simulink model "BacklashImplemented"  (R2018a)
settings: Solver=FixedStepDiscrete  StartTime=0.0  StopTime=10.0  RelTol=1e-3
settings Model: Creator=Laxman  LastModifiedBy=Laxman

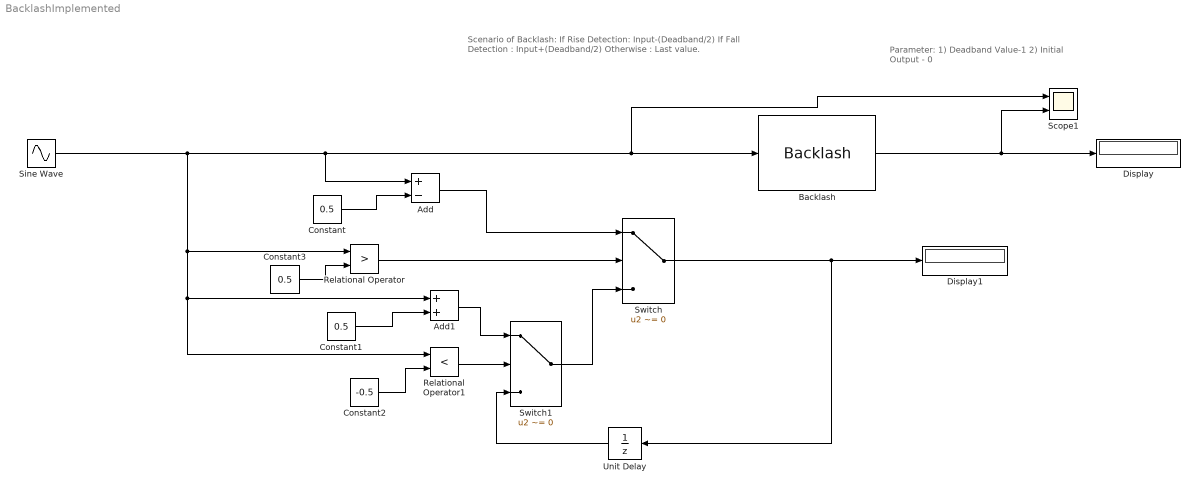
== system BacklashImplemented ==
  note: Parameter: 1) Deadband Value-1
      | 2) Initial Output - 0
  note: Scenario of Backlash:
      | If Rise Detection: Input-(Deadband/2)
      | If Fall Detection : Input+(Deadband/2)
      | Otherwise : Last value.
  Add : Sum  Inputs=+-
  Add1 : Sum
  Backlash : Backlash
  Constant : Constant  Value=0.5
  Constant1 : Constant  Value=0.5
  Constant2 : Constant  Value=-0.5
  Constant3 : Constant  Value=0.5
  Display : Display
  Display1 : Display
  Relational Operator : RelationalOperator  Operator=>  OutDataTypeStr=boolean  RndMeth=Simplest
  Relational Operator1 : RelationalOperator  Operator=<  OutDataTypeStr=boolean  RndMeth=Simplest
  Scope1 : Scope  NumInputPorts=2
  Sine Wave : Sin  SampleTime=0
  Switch : Switch  Criteria=u2 ~= 0
  Switch1 : Switch  Criteria=u2 ~= 0
  Unit Delay : UnitDelay  SampleTime=-1
  wires:
  Backlash/1 -> Scope1/2, Display/1
  Sine Wave/1 -> Add1/1, Relational Operator1/1, Relational Operator/1, Add/1, Scope1/1, Backlash/1
  Relational Operator/1 -> Switch/2
  Constant/1 -> Add/2
  Add/1 -> Switch/1
  Switch1/1 -> Switch/3
  Relational Operator1/1 -> Switch1/2
  Add1/1 -> Switch1/1
  Constant1/1 -> Add1/2
  Switch/1 -> Unit Delay/1, Display1/1
  Constant2/1 -> Relational Operator1/2
  Constant3/1 -> Relational Operator/2
  Unit Delay/1 -> Switch1/3
